simulink model "Cruise_Control"  (R2021a)
settings: Solver=VariableStepAuto  StartTime=0.0  StopTime=100  RelTol=1e-3
libraries: mpcadaslib x1
settings Model: Creator=91839  LastModifiedBy=91839

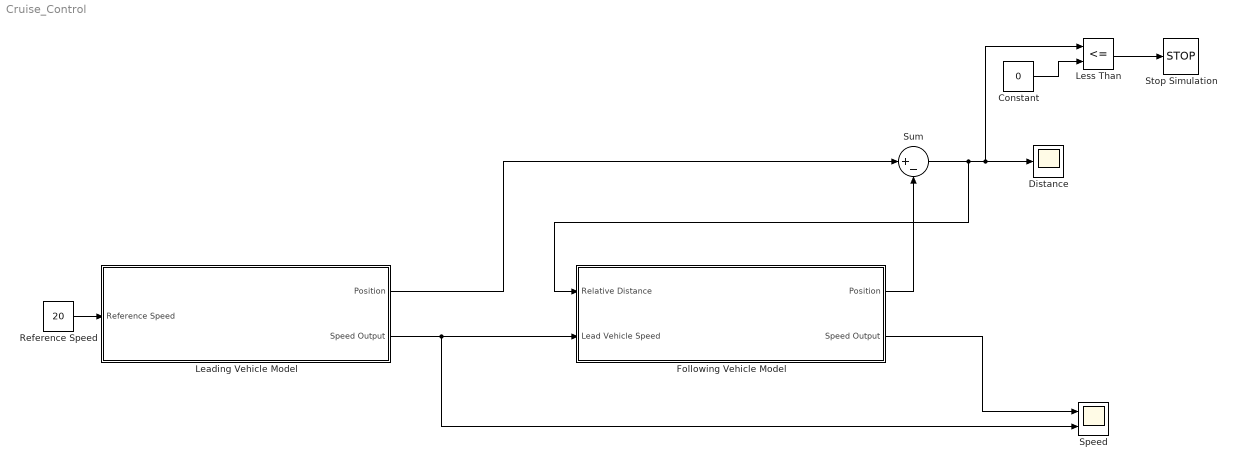
== system Cruise_Control ==
  Constant : Constant  Value=0
  Distance : Scope
  Following Vehicle Model : Subsystem  mask{Pos=0, Speed=30}
      mask prompts: Pos "Initial Position"; Speed "Initial Speed"
      mask TypeOptions Pos: Initial Position/Value
      mask TypeOptions Speed: Initial Speed/Value
  Leading Vehicle Model : Subsystem  mask{Pos=100, Speed=20}
      mask prompts: Pos "Initial Position"; Speed "Initial Speed"
      mask TypeOptions Pos: Initial Position/Value
      mask TypeOptions Speed: Initial Speed/Value
  Less Than : RelationalOperator  Operator=<=  OutDataTypeStr=boolean  RndMeth=Simplest
  Reference Speed : Constant  Value=20
  Speed : Scope  NumInputPorts=2
  Stop Simulation : Stop
  Sum : Sum  Inputs=|+-
  wires:
  Reference Speed/1 -> Leading Vehicle Model/1(Reference Speed)
  Leading Vehicle Model/2(Speed Output) -> Following Vehicle Model/2(Lead Vehicle Speed), Speed/2
  Following Vehicle Model/2(Speed Output) -> Speed/1
  Leading Vehicle Model/1(Position) -> Sum/1
  Following Vehicle Model/1(Position) -> Sum/2
  Sum/1 -> Following Vehicle Model/1(Relative Distance), Less Than/1, Distance/1
  Constant/1 -> Less Than/2
  Less Than/1 -> Stop Simulation/1

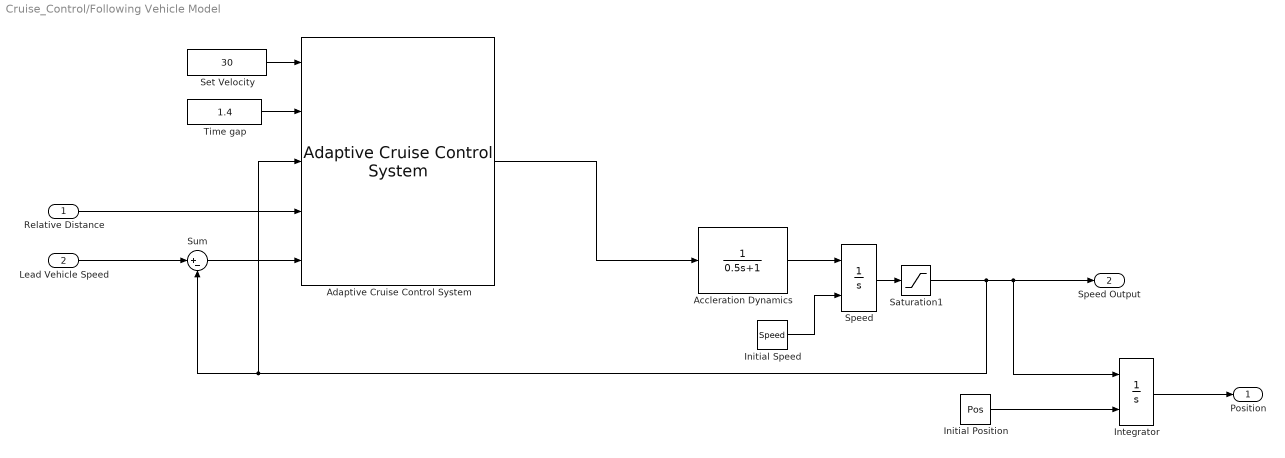
== system Cruise_Control/Following Vehicle Model ==
  Relative Distance : Inport
  Lead Vehicle Speed : Inport  Port=2
  Accleration Dynamics : TransferFcn  Denominator=[0.5 1]
  Adaptive Cruise Control System : mpcadaslib/Adaptive Cruise Control System  EgoModel=tf(1,[0.5,1,0])  InitialEgoVelocity=20  DefaultSpacing=10  MaxVelocity=50  MinAcceleration=-3  amin_ext=off  MaxAcceleration=2  amax_ext=off  Ts=0.1  PredictionHorizon=30  ControllerBehavior=0.5  suboptimal=off  maxiter=10  datatypeopt=double  optmode=off  trackmode=off
  Initial Position : Constant  Value=Pos
  Initial Speed : Constant  Value=Speed
  Integrator : Integrator  InitialConditionSource=external
  Saturation1 : Saturate  UpperLimit=inf  LowerLimit=0
  Set Velocity : Constant  Value=30
  Speed : Integrator  InitialConditionSource=external
  Sum : Sum  Inputs=|+-
  Time gap : Constant  Value=1.4
  Position : Outport
  Speed Output : Outport  Port=2
  wires:
  Initial Position/1 -> Integrator/2
  Speed/1 -> Saturation1/1
  Lead Vehicle Speed/1 -> Sum/1
  Integrator/1 -> Position/1
  Initial Speed/1 -> Speed/2
  Saturation1/1 -> Integrator/1, Speed Output/1, Adaptive Cruise Control System/3, Sum/2
  Adaptive Cruise Control System/1 -> Accleration Dynamics/1
  Accleration Dynamics/1 -> Speed/1
  Sum/1 -> Adaptive Cruise Control System/5
  Relative Distance/1 -> Adaptive Cruise Control System/4
  Set Velocity/1 -> Adaptive Cruise Control System/1
  Time gap/1 -> Adaptive Cruise Control System/2

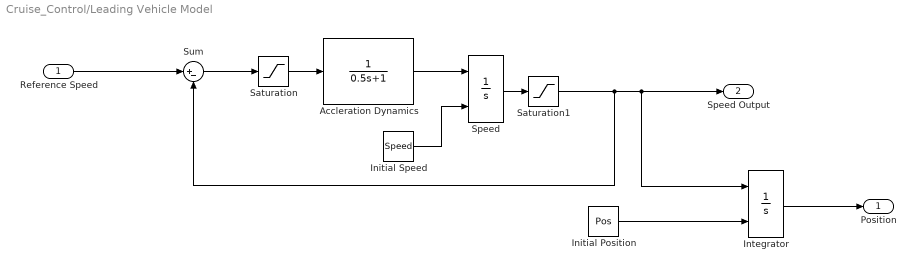
== system Cruise_Control/Leading Vehicle Model ==
  Reference Speed : Inport
  Accleration Dynamics : TransferFcn  Denominator=[0.5 1]
  Initial Position : Constant  Value=Pos
  Initial Speed : Constant  Value=Speed
  Integrator : Integrator  InitialConditionSource=external
  Saturation : Saturate  UpperLimit=2  LowerLimit=-3
  Saturation1 : Saturate  UpperLimit=inf  LowerLimit=0
  Speed : Integrator  InitialConditionSource=external
  Sum : Sum  Inputs=|+-
  Position : Outport
  Speed Output : Outport  Port=2
  wires:
  Sum/1 -> Saturation/1
  Accleration Dynamics/1 -> Speed/1
  Saturation/1 -> Accleration Dynamics/1
  Saturation1/1 -> Sum/2, Speed Output/1, Integrator/1
  Initial Speed/1 -> Speed/2
  Integrator/1 -> Position/1
  Reference Speed/1 -> Sum/1
  Speed/1 -> Saturation1/1
  Initial Position/1 -> Integrator/2
